simulink model "openMHA_test_FFT_to_gain"  (R2020b)
settings: Solver=VariableStepAuto  StartTime=0.0  StopTime=stop_time  RelTol=1e-3
InitFcn:
  | test_FFT_to_gain_init
StopFcn:
  | test_FFT_to_gain_stop
values from neighbouring files (symbols this model uses):
  band_edges = [band_edges mirrored_band_edges]    [test_FFT_to_gain_init.m]    (also in test_db_lookup_gain_fpga_init.m = calculate_band_edges(ef, num_bins, binwidth, num_bands); test_db_lookup_init.m = calculate_band_edges(ef, num_bins, binwidth, num_bands); test_gaintable_init.m = calculate_band_edges(ef, num_bins, binwidth, num_bands); test_init.m = calculate_band_edges(ef, num_bins, binwidth, num_bands))
  buf_a = 65.*ones(num_bands,1)    [test_FFT_to_gain_init.m]    (also in test_ar_filter_dualport_init.m; test_db_ar_gaintable_init.m)
  delay_memory_size = 2^system_delay_memory    [test_FFT_to_gain_init.m]    (also in test_state_gainapp_cbuf_init.m)
  FFTsize = 256    [test_FFT_to_gain_init.m]    (also in test_ar_filter_gaintable_init.m; test_db_ar_gaintable_init.m; test_db_lookup_gain_fpga_init.m; test_db_lookup_init.m)
  gainapp_dp_memory = log2(num_bands) + 1    [test_FFT_to_gain_init.m]    (also in test_state_gainapp_cbuf_init.m)
  num_bands = 8    [calculate_gaintable.m]    (also in test_FFT_to_gain_init.m = 2; test_ar_filter_dualport_init.m = 2; test_db_ar_gaintable_init.m = 2; test_db_lookup_gain_fpga_init.m = 9)
  num_bins = FFTsize/2 + 1    (= 129)    [test_FFT_to_gain_init.m]    (also in test_ar_filter_gaintable_init.m; test_db_ar_gaintable_init.m; test_db_lookup_gain_fpga_init.m; test_db_lookup_init.m)
  system_delay = 6 + max(band_sizes)    [test_FFT_to_gain_init.m]    (also in test_state_gainapp_cbuf_init.m = max(band_sizes))
  table_length = length(gtdata)    [calculate_gaintable.m]    (also in test_FFT_to_gain_init.m; test_ar_filter_gaintable_init.m; test_db_ar_gaintable_init.m; test_db_lookup_gain_fpga_init.m)
  X_high = 93    [test_FFT_to_gain_init.m]    (also in test_ar_filter_gaintable_init.m = 95; test_db_ar_gaintable_init.m; test_db_lookup_gain_fpga_init.m = 95; test_db_lookup_init.m = 95)
  xIn = [4.65661287308e-10 5.23868948221e-10 5.82076609135e-10 6.40284270048e-10 6.98491930962e-10 7.56699591875e-10 8.14907252789e-10 8.73114913702e-10 9.31322574615e-10 1.04773789644e-09 1.16415321827e-09 1.2805685401e-09 ... (256 elements, 1x256)]    [openMHA_test_db_lookup_gain_Programmable Look-Up Table_init.mat]    (also in openMHA_test_db_lookup_gain_Programmable Lookup Table dB_init.mat = [4.65661287308e-10 4.72937244922e-10 4.80213202536e-10 4.874)
libraries: dspsrcs4 x9, hdlsllib x8, simulink x4, FPGA_Open_Speech_Tools x3
(part 1 of 2)
settings Model: Creator=t96f346  LastModifiedBy=t96f346

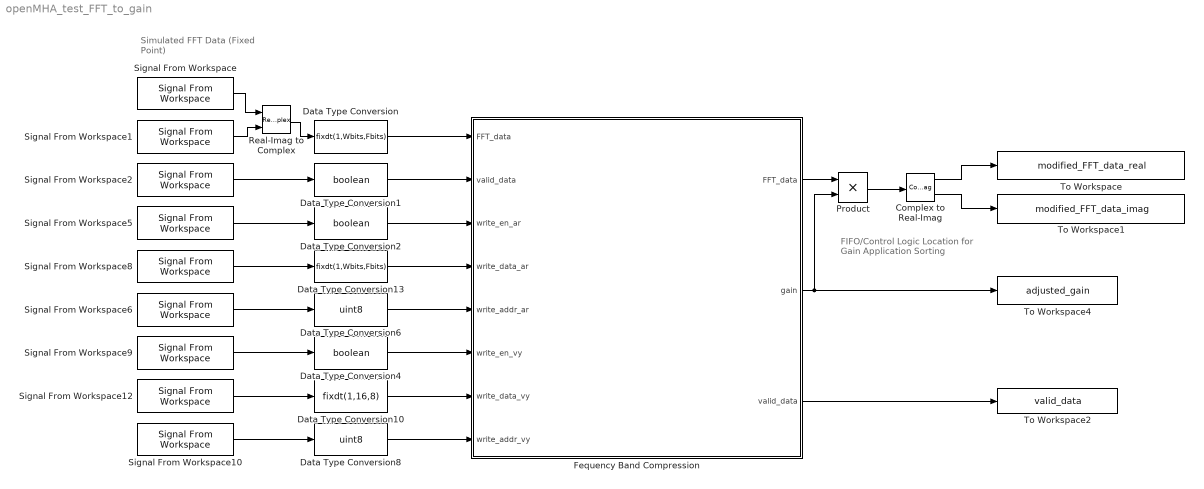
== system openMHA_test_FFT_to_gain ==
  note: Simulated FFT Data
      | (Fixed Point)
  note: FIFO/Control Logic Location for Gain Application Sorting
  Complex to Real-Imag : ComplexToRealImag
  Data Type Conversion : DataTypeConversion  OutDataTypeStr=fixdt(1,Wbits,Fbits)
  Data Type Conversion1 : DataTypeConversion  OutDataTypeStr=boolean
  Data Type Conversion10 : DataTypeConversion  OutDataTypeStr=fixdt(1,16,8)
  Data Type Conversion13 : DataTypeConversion  OutDataTypeStr=fixdt(1,Wbits,Fbits)
  Data Type Conversion2 : DataTypeConversion  OutDataTypeStr=boolean
  Data Type Conversion4 : DataTypeConversion  OutDataTypeStr=boolean
  Data Type Conversion6 : DataTypeConversion  OutDataTypeStr=uint8
  Data Type Conversion8 : DataTypeConversion  OutDataTypeStr=uint8
  Fequency Band Compression : Subsystem
  Product : Product
  Real-Imag to Complex : RealImagToComplex
  Signal From Workspace : dspsrcs4/Signal From Workspace  X=FFT_data_real  Ts=1  nsamps=1  OutputAfterFinalValue=Setting to zero  ignoreOrWarnInputAndFrameLengths=off  OutputFrames=off
  Signal From Workspace1 : dspsrcs4/Signal From Workspace  X=FFT_data_imag  Ts=1  nsamps=1  OutputAfterFinalValue=Setting to zero  ignoreOrWarnInputAndFrameLengths=off  OutputFrames=off
  Signal From Workspace10 : dspsrcs4/Signal From Workspace  X=write_addr_vy  Ts=1  nsamps=1  OutputAfterFinalValue=Setting to zero  ignoreOrWarnInputAndFrameLengths=off  OutputFrames=off
  Signal From Workspace12 : dspsrcs4/Signal From Workspace  X=write_data_vy  Ts=1  nsamps=1  OutputAfterFinalValue=Setting to zero  ignoreOrWarnInputAndFrameLengths=off  OutputFrames=off
  Signal From Workspace2 : dspsrcs4/Signal From Workspace  X=valid_data  Ts=1  nsamps=1  OutputAfterFinalValue=Setting to zero  ignoreOrWarnInputAndFrameLengths=off  OutputFrames=off
  Signal From Workspace5 : dspsrcs4/Signal From Workspace  X=write_en_ar  Ts=1  nsamps=1  OutputAfterFinalValue=Setting to zero  ignoreOrWarnInputAndFrameLengths=off  OutputFrames=off
  Signal From Workspace6 : dspsrcs4/Signal From Workspace  X=write_addr_ar  Ts=1  nsamps=1  OutputAfterFinalValue=Setting to zero  ignoreOrWarnInputAndFrameLengths=off  OutputFrames=off
  Signal From Workspace8 : dspsrcs4/Signal From Workspace  X=write_data_ar  Ts=1  nsamps=1  OutputAfterFinalValue=Setting to zero  ignoreOrWarnInputAndFrameLengths=off  OutputFrames=off
  Signal From Workspace9 : dspsrcs4/Signal From Workspace  X=write_en_vy  Ts=1  nsamps=1  OutputAfterFinalValue=Setting to zero  ignoreOrWarnInputAndFrameLengths=off  OutputFrames=off
  To Workspace : ToWorkspace  VariableName=modified_FFT_data_real  SampleTime=-1
      settings: Save2DSignal=2-D array (concatenate along first dimension)
  To Workspace1 : ToWorkspace  VariableName=modified_FFT_data_imag  SampleTime=-1
      settings: Save2DSignal=2-D array (concatenate along first dimension)
  To Workspace2 : ToWorkspace  VariableName=valid_data  SampleTime=-1
      settings: Save2DSignal=2-D array (concatenate along first dimension)
  To Workspace4 : ToWorkspace  VariableName=adjusted_gain  SampleTime=-1
      settings: Save2DSignal=2-D array (concatenate along first dimension)
  wires:
  Real-Imag to Complex/1 -> Data Type Conversion/1
  Signal From Workspace1/1 -> Real-Imag to Complex/2
  Signal From Workspace/1 -> Real-Imag to Complex/1
  Product/1 -> Complex to Real-Imag/1
  Complex to Real-Imag/2 -> To Workspace1/1
  Complex to Real-Imag/1 -> To Workspace/1
  Data Type Conversion/1 -> Fequency Band Compression/1(FFT_data)
  Signal From Workspace2/1 -> Data Type Conversion1/1
  Signal From Workspace12/1 -> Data Type Conversion10/1
  Signal From Workspace8/1 -> Data Type Conversion13/1
  Signal From Workspace10/1 -> Data Type Conversion8/1
  Signal From Workspace9/1 -> Data Type Conversion4/1
  Signal From Workspace6/1 -> Data Type Conversion6/1
  Signal From Workspace5/1 -> Data Type Conversion2/1
  Data Type Conversion2/1 -> Fequency Band Compression/3(write_en_ar)
  Data Type Conversion13/1 -> Fequency Band Compression/4(write_data_ar)
  Data Type Conversion6/1 -> Fequency Band Compression/5(write_addr_ar)
  Data Type Conversion4/1 -> Fequency Band Compression/6(write_en_vy)
  Data Type Conversion10/1 -> Fequency Band Compression/7(write_data_vy)
  Data Type Conversion8/1 -> Fequency Band Compression/8(write_addr_vy)
  Fequency Band Compression/2(gain) -> Product/2, To Workspace4/1
  Data Type Conversion1/1 -> Fequency Band Compression/2(valid_data)
  Fequency Band Compression/1("FFT_data ") -> Product/1
  Fequency Band Compression/3("valid_data ") -> To Workspace2/1

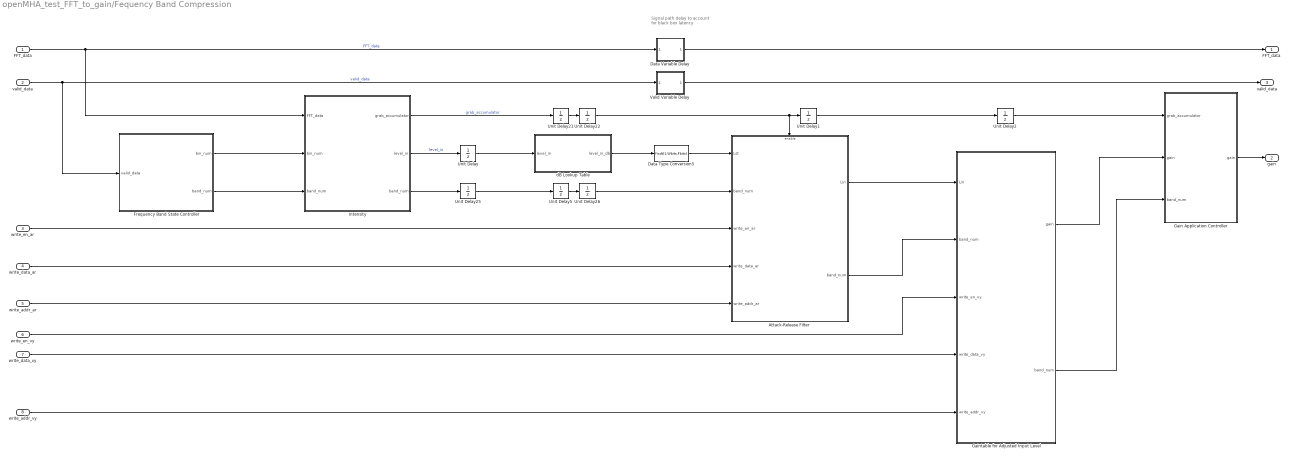
== system openMHA_test_FFT_to_gain/Fequency Band Compression ==
  note: Signal path delay to account for black box latency
  FFT_data : Inport
  valid_data : Inport  Port=2
  write_en_ar : Inport  Port=3
  write_data_ar : Inport  Port=4
  write_addr_ar : Inport  Port=5
  write_en_vy : Inport  Port=6
  write_data_vy : Inport  Port=7
  write_addr_vy : Inport  Port=8
  Attack-Release Filter : Subsystem
  Data Type Conversion5 : DataTypeConversion  OutDataTypeStr=fixdt(1,Wbits,Fbits)
  Data Variable Delay : Subsystem
  Frequency Band State Controller : Subsystem
  Gain Application Controller : Subsystem
  Gaintable for Adjusted Input Level : Subsystem
  Intensity : Subsystem
  Unit Delay{,1..2,5,21..22,25..26} (8 alike) : UnitDelay  SampleTime=-1  HasFrameUpgradeWarning=on
  Valid Variable Delay : Subsystem
  dB Lookup Table : Subsystem
  "FFT_data " : Outport
  gain : Outport  Port=2
  "valid_data " : Outport  Port=3
  wires:
  Gaintable for Adjusted Input Level/1(gain) -> Gain Application Controller/2(gain)
  Intensity/2(level_in) -> Unit Delay/1  "level_in"
  valid_data/1 -> Valid Variable Delay/1(data_in), Frequency Band State Controller/1(valid_data)  "valid_data"
  Intensity/1(grab_accumulator) -> Unit Delay21/1  "grab_accumulator"
  FFT_data/1 -> Data Variable Delay/1(data_in), Intensity/1(FFT_data)  "FFT_data"
  Intensity/3("band_num ") -> Unit Delay25/1
  Unit Delay25/1 -> Unit Delay5/1
  Valid Variable Delay/1(rd_dout) -> "valid_data "/1
  Data Variable Delay/1(rd_dout) -> "FFT_data "/1
  Data Type Conversion5/1 -> Attack-Release Filter/1(Lst)
  dB Lookup Table/1(level_in_db) -> Data Type Conversion5/1
  Unit Delay/1 -> dB Lookup Table/1(level_in)
  Unit Delay5/1 -> Unit Delay26/1
  Unit Delay26/1 -> Attack-Release Filter/2(band_num)
  Attack-Release Filter/1(Lin) -> Gaintable for Adjusted Input Level/1(Lin)
  Attack-Release Filter/2("band_num ") -> Gaintable for Adjusted Input Level/2(band_num)
  Frequency Band State Controller/1(bin_num) -> Intensity/2(bin_num)
  Frequency Band State Controller/2(band_num) -> Intensity/3(band_num)
  Unit Delay21/1 -> Unit Delay22/1
  Unit Delay22/1 -> Attack-Release Filter/Enable, Unit Delay1/1
  write_en_ar/1 -> Attack-Release Filter/3(write_en_ar)
  write_data_ar/1 -> Attack-Release Filter/4(write_data_ar)
  write_addr_ar/1 -> Attack-Release Filter/5(write_addr_ar)
  write_en_vy/1 -> Gaintable for Adjusted Input Level/3(write_en_vy)
  write_data_vy/1 -> Gaintable for Adjusted Input Level/4(write_data_vy)
  write_addr_vy/1 -> Gaintable for Adjusted Input Level/5(write_addr_vy)
  Gaintable for Adjusted Input Level/2("band_num ") -> Gain Application Controller/3(band_num)
  Unit Delay1/1 -> Unit Delay2/1
  Unit Delay2/1 -> Gain Application Controller/1(grab_accumulator)
  Gain Application Controller/1("gain ") -> gain/1

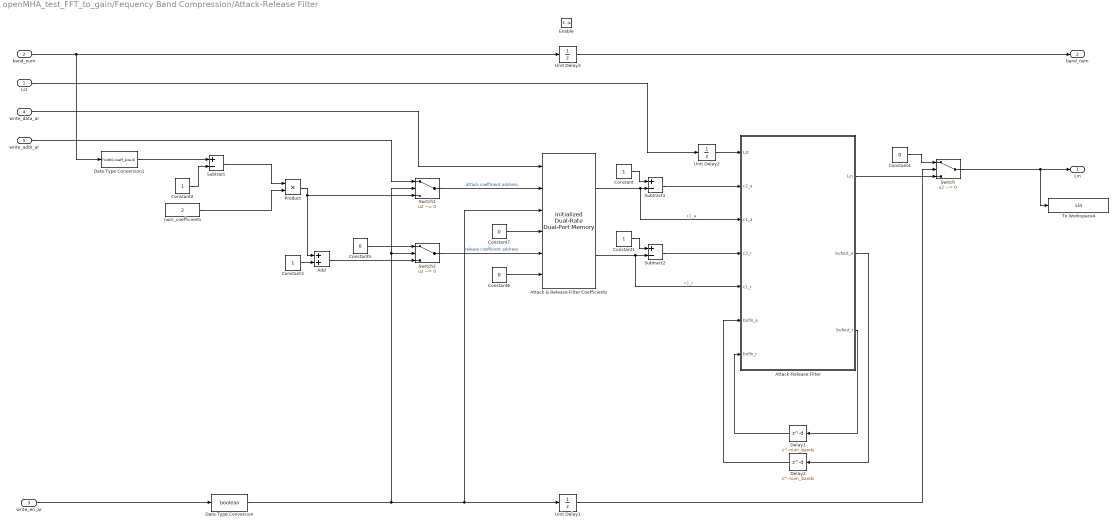
== system openMHA_test_FFT_to_gain/Fequency Band Compression/Attack-Release Filter ==
  Lst : Inport
  band_num : Inport  Port=2
  write_en_ar : Inport  Port=3
  write_data_ar : Inport  Port=4
  write_addr_ar : Inport  Port=5
  Enable : EnablePort
  Add : Sum
  Attack & Release Filter Coefficients : FPGA_Open_Speech_Tools/Initialized Dual-Rate Dual-Port Memory  ram_size=coeff_size  Table_Init=ar_coeffs
      settings: SourceProductName=FPGA Open Speech Tools
  Attack-Release Filter : Subsystem
  Constant : Constant  OutDataTypeStr=fixdt(1,Wbits,Fbits)  SampleTime=-1
  Constant1 : Constant  OutDataTypeStr=fixdt(1,Wbits,Fbits)  SampleTime=-1
  Constant2 : Constant  OutDataTypeStr=fixdt(0,coeff_size,0)  SampleTime=-1
  Constant3 : Constant  OutDataTypeStr=uint8  SampleTime=-1
  Constant4 : Constant  Value=0  OutDataTypeStr=fixdt(1,Wbits,Fbits)  SampleTime=-1
  Constant5 : Constant  Value=0  OutDataTypeStr=uint8  SampleTime=-1
  Constant6 : Constant  Value=0  OutDataTypeStr=boolean  SampleTime=-1
  Constant7 : Constant  Value=0  OutDataTypeStr=fixdt(1,Wbits,Fbits)  SampleTime=-1
  Data Type Conversion : DataTypeConversion  OutDataTypeStr=boolean
  Data Type Conversion1 : DataTypeConversion  OutDataTypeStr=fixdt(0,coeff_size,0)
  Delay1 : Delay  DelayLength=num_bands  InitialCondition=buf_a  UseCircularBuffer=on
  Delay2 : Delay  DelayLength=num_bands  InitialCondition=buf_a  UseCircularBuffer=on
  Product : Product  OutDataTypeStr=fixdt(0,coeff_size,0)
  Subtract : Sum  Inputs=+-  OutDataTypeStr=fixdt(0,coeff_size,0)
  Subtract1 : Sum  Inputs=+-  OutDataTypeStr=fixdt(1,Wbits,Fbits)
  Subtract2 : Sum  Inputs=+-  OutDataTypeStr=fixdt(1,Wbits,Fbits)
  Switch : Switch  Criteria=u2 ~= 0  OutDataTypeStr=fixdt(1,Wbits,Fbits)
  Switch1 : Switch  Criteria=u2 ~= 0  OutDataTypeStr=Inherit: Inherit via back propagation
  Switch2 : Switch  Criteria=u2 ~= 0  OutDataTypeStr=uint8
  To Workspace4 : ToWorkspace  VariableName=Lin  SampleTime=-1
      settings: Save2DSignal=2-D array (concatenate along first dimension)
  Unit Delay1 : UnitDelay  SampleTime=-1  HasFrameUpgradeWarning=on
  Unit Delay2 : UnitDelay  InitialCondition=65  SampleTime=-1  HasFrameUpgradeWarning=on
  Unit Delay3 : UnitDelay  InitialCondition=1  SampleTime=-1  HasFrameUpgradeWarning=on
  num_coefficients : Constant  Value=2  OutDataTypeStr=uint8  SampleTime=-1
  Lin : Outport
  "band_num " : Outport  Port=2
  wires:
  Constant4/1 -> Switch/1
  Constant2/1 -> Subtract/2
  Attack-Release Filter/2(bufout_a) -> Delay2/1
  Delay1/1 -> Attack-Release Filter/7(bufin_r)
  Constant6/1 -> Attack & Release Filter Coefficients/6
  Constant3/1 -> Add/2
  Switch1/1 -> Attack & Release Filter Coefficients/2  "attack coefficient address"
  Constant5/1 -> Switch2/1
  Subtract1/1 -> Attack-Release Filter/2(c2_a)
  num_coefficients/1 -> Product/2
  Attack & Release Filter Coefficients/2 -> Attack-Release Filter/5(c1_r), Subtract2/2  "c1_r"
  Constant7/1 -> Attack & Release Filter Coefficients/4
  Attack-Release Filter/1(Lin) -> Switch/3
  Subtract/1 -> Product/1
  Unit Delay2/1 -> Attack-Release Filter/1(Lst)
  Data Type Conversion1/1 -> Subtract/1
  Constant/1 -> Subtract1/1
  Constant1/1 -> Subtract2/1
  Switch2/1 -> Attack & Release Filter Coefficients/5  "release coefficient address"
  Product/1 -> Add/1, Switch1/3
  Data Type Conversion/1 -> Switch1/2, Switch2/2, Unit Delay1/1, Attack & Release Filter Coefficients/3
  Unit Delay1/1 -> Switch/2
  Subtract2/1 -> Attack-Release Filter/4(c2_r)
  Attack-Release Filter/3(bufout_r) -> Delay1/1
  Delay2/1 -> Attack-Release Filter/6(bufin_a)
  Add/1 -> Switch2/3
  Attack & Release Filter Coefficients/1 -> Attack-Release Filter/3(c1_a), Subtract1/2  "c1_a"
  band_num/1 -> Data Type Conversion1/1, Unit Delay3/1
  Lst/1 -> Unit Delay2/1
  write_data_ar/1 -> Attack & Release Filter Coefficients/1
  write_addr_ar/1 -> Switch1/1
  Switch/1 -> To Workspace4/1, Lin/1
  Unit Delay3/1 -> "band_num "/1
  write_en_ar/1 -> Data Type Conversion/1

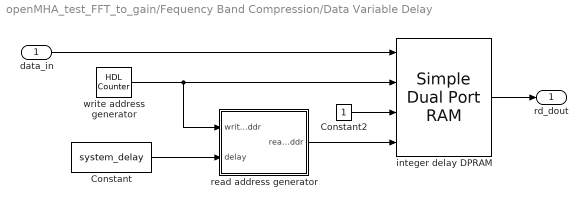
== system openMHA_test_FFT_to_gain/Fequency Band Compression/Data Variable Delay ==
  data_in : Inport
  Constant : Constant  Value=system_delay  OutDataTypeStr=uint8  SampleTime=-1
  Constant2 : Constant  OutDataTypeStr=Inherit: Inherit via back propagation  SampleTime=-1
  integer delay DPRAM : hdlsllib/HDL RAMs/Simple Dual Port RAM  ram_size=system_delay_memory
      settings: SourceProductBaseCode=SL
  read address generator : Subsystem
  write address generator : hdlsllib/Sources/HDL Counter  CountType=Count limited  CountInit=0  CountStep=1  CountMax=delay_memory_size - 1  CountFromType=Initial value  CountFrom=0  CountResetPort=off  CountLoadPort=off  CountEnbPort=off  CountDirPort=off  CountDataType=Unsigned  CountWordLen=system_delay_memory  CountFracLen=0  CountSampTime=-1
  rd_dout : Outport
  wires:
  Constant2/1 -> integer delay DPRAM/3
  write address generator/1 -> integer delay DPRAM/2, read address generator/1(write_addr)
  integer delay DPRAM/1 -> rd_dout/1
  Constant/1 -> read address generator/2(delay)
  data_in/1 -> integer delay DPRAM/1
  read address generator/1(read_addr) -> integer delay DPRAM/4

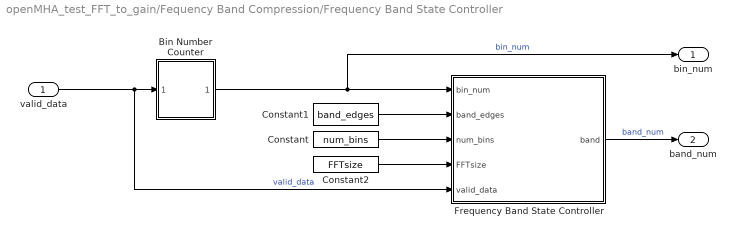
== system openMHA_test_FFT_to_gain/Fequency Band Compression/Frequency Band State Controller ==
  valid_data : Inport
  Bin Number Counter : Subsystem
  Constant : Constant  Value=num_bins  SampleTime=-1
  Constant1 : Constant  Value=band_edges  SampleTime=-1
  Constant2 : Constant  Value=FFTsize  SampleTime=-1
  Frequency Band State Controller : MATLAB Function  TreatAsAtomicUnit=on
  bin_num : Outport
  band_num : Outport  Port=2
  wires:
  Bin Number Counter/1(bin_num) -> bin_num/1, Frequency Band State Controller/1(bin_num)  "bin_num"
  Constant2/1 -> Frequency Band State Controller/4(FFTsize)
  valid_data/1 -> Frequency Band State Controller/5(valid_data), Bin Number Counter/1(valid_data)  "valid_data"
  Constant/1 -> Frequency Band State Controller/3(num_bins)
  Constant1/1 -> Frequency Band State Controller/2(band_edges)
  Frequency Band State Controller/1(band) -> band_num/1  "band_num"

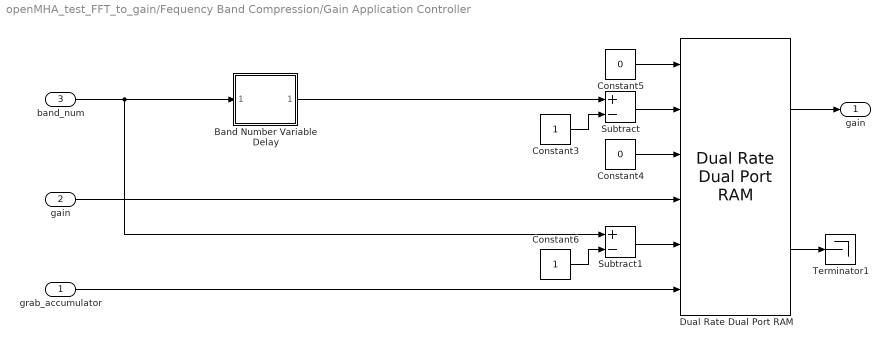
== system openMHA_test_FFT_to_gain/Fequency Band Compression/Gain Application Controller ==
  grab_accumulator : Inport
  gain : Inport  Port=2
  band_num : Inport  Port=3
  Band Number Variable Delay : Subsystem
  Constant3 : Constant  SampleTime=-1
  Constant4 : Constant  Value=0  OutDataTypeStr=boolean  SampleTime=-1
  Constant5 : Constant  Value=0  OutDataTypeStr=fixdt(1,16,8)  SampleTime=-1
  Constant6 : Constant  SampleTime=-1
  Dual Rate Dual Port RAM : hdlsllib/HDL RAMs/Dual Rate Dual Port RAM  ram_size=gainapp_dp_memory
      settings: SourceProductBaseCode=SL
  Subtract : Sum  Inputs=+-  OutMin=[0]  OutMax=[2^gainapp_dp_memory-1]  OutDataTypeStr=fixdt(0,gainapp_dp_memory)
  Subtract1 : Sum  Inputs=+-  OutMin=[0]  OutMax=[2^gainapp_dp_memory-1]  OutDataTypeStr=fixdt(0,gainapp_dp_memory)
  Terminator1 : Terminator
  "gain " : Outport
  wires:
  Dual Rate Dual Port RAM/1 -> "gain "/1
  Constant5/1 -> Dual Rate Dual Port RAM/1
  Constant6/1 -> Subtract1/2
  Constant3/1 -> Subtract/2
  Constant4/1 -> Dual Rate Dual Port RAM/3
  grab_accumulator/1 -> Dual Rate Dual Port RAM/6
  Subtract1/1 -> Dual Rate Dual Port RAM/5
  Band Number Variable Delay/1(rd_dout) -> Subtract/1
  Dual Rate Dual Port RAM/2 -> Terminator1/1
  gain/1 -> Dual Rate Dual Port RAM/4
  Subtract/1 -> Dual Rate Dual Port RAM/2
  band_num/1 -> Band Number Variable Delay/1(data_in), Subtract1/1

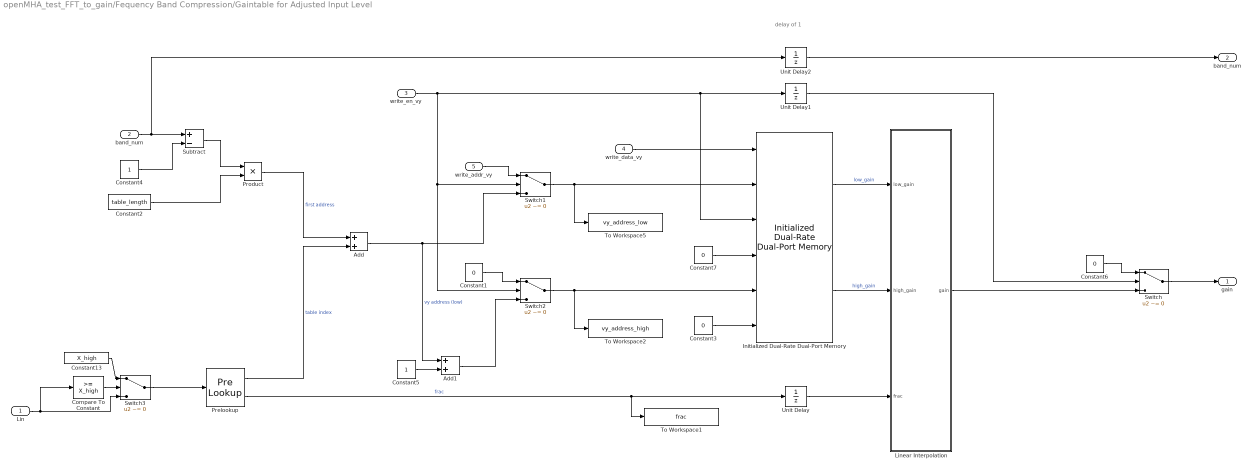
== system openMHA_test_FFT_to_gain/Fequency Band Compression/Gaintable for Adjusted Input Level ==
  note: delay of 1
  Lin : Inport
  band_num : Inport  Port=2
  write_en_vy : Inport  Port=3
  write_data_vy : Inport  Port=4
  write_addr_vy : Inport  Port=5
  Add : Sum  OutDataTypeStr=uint8
  Add1 : Sum  OutDataTypeStr=uint8
  Compare To Constant : simulink/Logic and Bit Operations/Compare To Constant  relop=>=  const=X_high  OutDataTypeStr=boolean
  Constant1 : Constant  Value=0  OutDataTypeStr=uint8  SampleTime=-1
  Constant13 : Constant  Value=X_high  OutDataTypeStr=fixdt(1,Wbits, Fbits)  SampleTime=-1
  Constant2 : Constant  Value=table_length  OutDataTypeStr=uint8  SampleTime=-1
  Constant3 : Constant  Value=0  OutDataTypeStr=boolean  SampleTime=-1
  Constant4 : Constant  OutDataTypeStr=uint8  SampleTime=-1
  Constant5 : Constant  OutDataTypeStr=uint8  SampleTime=-1
  Constant6 : Constant  Value=0  OutDataTypeStr=fixdt(1,16,8)  SampleTime=-1
  Constant7 : Constant  Value=0  OutDataTypeStr=fixdt(1,16,8)  SampleTime=-1
  Initialized Dual-Rate Dual-Port Memory : FPGA_Open_Speech_Tools/Initialized Dual-Rate Dual-Port Memory  ram_size=RAM_size  Table_Init=vy
      settings: SourceProductName=FPGA Open Speech Tools
  Linear Interpolation : Subsystem
  Prelookup : PreLookup  BreakpointsData=input_levels_db  IndexSearchMethod=Evenly spaced points  UseLastBreakpoint=on  DiagnosticForOutOfRangeInput=Error  IndexDataTypeStr=uint8
  Product : Product  OutDataTypeStr=Inherit: Same as first input
  Subtract : Sum  Inputs=+-
  Switch : Switch  Criteria=u2 ~= 0  OutDataTypeStr=fixdt(1,16,8)
  Switch1 : Switch  Criteria=u2 ~= 0  OutDataTypeStr=uint8
  Switch2 : Switch  Criteria=u2 ~= 0  OutDataTypeStr=uint8
  Switch3 : Switch  Criteria=u2 ~= 0
  To Workspace1 : ToWorkspace  VariableName=frac  SampleTime=-1
      settings: Save2DSignal=2-D array (concatenate along first dimension)
  To Workspace2 : ToWorkspace  VariableName=vy_address_high  SampleTime=-1
      settings: Save2DSignal=2-D array (concatenate along first dimension)
  To Workspace5 : ToWorkspace  VariableName=vy_address_low  SampleTime=-1
      settings: Save2DSignal=2-D array (concatenate along first dimension)
  Unit Delay : UnitDelay  SampleTime=-1  HasFrameUpgradeWarning=on
  Unit Delay1 : UnitDelay  InitialCondition=1  SampleTime=-1  HasFrameUpgradeWarning=on
  Unit Delay2 : UnitDelay  InitialCondition=1  SampleTime=-1  HasFrameUpgradeWarning=on
  gain : Outport
  "band_num " : Outport  Port=2
  wires:
  write_data_vy/1 -> Initialized Dual-Rate Dual-Port Memory/1
  Unit Delay/1 -> Linear Interpolation/3(frac)
  Unit Delay1/1 -> Switch/2
  Compare To Constant/1 -> Switch3/2
  Switch/1 -> gain/1
  band_num/1 -> Unit Delay2/1, Subtract/1
  Constant6/1 -> Switch/1
  Add/1 -> Switch1/3, Add1/1  "vy address (low)"
  Linear Interpolation/1(gain) -> Switch/3
  Initialized Dual-Rate Dual-Port Memory/2 -> Linear Interpolation/2(high_gain)  "high_gain"
  Switch1/1 -> Initialized Dual-Rate Dual-Port Memory/2, To Workspace5/1
  write_en_vy/1 -> Initialized Dual-Rate Dual-Port Memory/3, Unit Delay1/1, Switch1/2, Switch2/2
  Constant5/1 -> Add1/2
  Prelookup/1 -> Add/2  "table index"
  Constant13/1 -> Switch3/1
  Add1/1 -> Switch2/3
  Initialized Dual-Rate Dual-Port Memory/1 -> Linear Interpolation/1(low_gain)  "low_gain"
  Switch2/1 -> Initialized Dual-Rate Dual-Port Memory/5, To Workspace2/1
  Constant4/1 -> Subtract/2
  Prelookup/2 -> To Workspace1/1, Unit Delay/1  "frac"
  Product/1 -> Add/1  "first address"
  Subtract/1 -> Product/1
  Lin/1 -> Compare To Constant/1, Switch3/3
  Constant2/1 -> Product/2
  Switch3/1 -> Prelookup/1
  write_addr_vy/1 -> Switch1/1
  Constant1/1 -> Switch2/1
  Constant3/1 -> Initialized Dual-Rate Dual-Port Memory/6
  Constant7/1 -> Initialized Dual-Rate Dual-Port Memory/4
  Unit Delay2/1 -> "band_num "/1

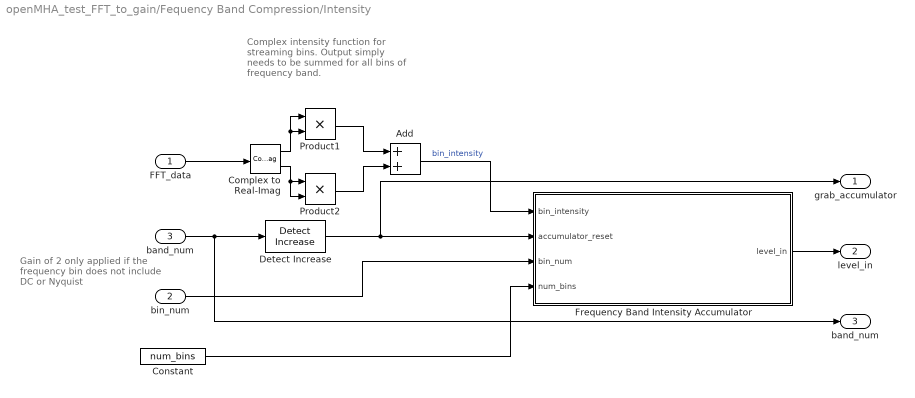
== system openMHA_test_FFT_to_gain/Fequency Band Compression/Intensity ==
  note: Complex intensity function for streaming bins. Output simply needs to be summed for all bins of frequency band.
  note: Gain of 2 only applied if the frequency bin does not include DC or Nyquist
  FFT_data : Inport
  bin_num : Inport  Port=2
  band_num : Inport  Port=3
  Add : Sum  OutDataTypeStr=fixdt(1,Wbits,Fbits)
  Complex to Real-Imag : ComplexToRealImag
  Constant : Constant  Value=num_bins  OutDataTypeStr=uint8  SampleTime=-1
  Detect Increase : simulink/Logic and Bit Operations/Detect Increase  vinit=1  OutDataTypeStr=boolean
  Frequency Band Intensity Accumulator : MATLAB Function  TreatAsAtomicUnit=on
  Product1 : Product  OutDataTypeStr=fixdt(1,Wbits,Fbits)
  Product2 : Product  OutDataTypeStr=fixdt(1,Wbits,Fbits)
  grab_accumulator : Outport  VectorParamsAs1DForOutWhenUnconnected=off
  level_in : Outport  Port=2
  "band_num " : Outport  Port=3
  wires:
  Product2/1 -> Add/2
  Complex to Real-Imag/1 -> Product1/1, Product1/2
  Complex to Real-Imag/2 -> Product2/2, Product2/1
  Product1/1 -> Add/1
  Add/1 -> Frequency Band Intensity Accumulator/1(bin_intensity)  "bin_intensity"
  FFT_data/1 -> Complex to Real-Imag/1
  Frequency Band Intensity Accumulator/1(level_in) -> level_in/1
  band_num/1 -> Detect Increase/1, "band_num "/1
  Detect Increase/1 -> Frequency Band Intensity Accumulator/2(accumulator_reset), grab_accumulator/1
  bin_num/1 -> Frequency Band Intensity Accumulator/3(bin_num)
  Constant/1 -> Frequency Band Intensity Accumulator/4(num_bins)

== system openMHA_test_FFT_to_gain/Fequency Band Compression/Valid Variable Delay ==
  data_in : Inport
  Constant : Constant  Value=system_delay  OutDataTypeStr=uint8  SampleTime=-1
  Constant2 : Constant  OutDataTypeStr=Inherit: Inherit via back propagation  SampleTime=-1
  integer delay DPRAM : hdlsllib/HDL RAMs/Simple Dual Port RAM  ram_size=system_delay_memory
      settings: SourceProductBaseCode=SL
  read address generator : Subsystem
  write address generator : hdlsllib/Sources/HDL Counter  CountType=Count limited  CountInit=0  CountStep=1  CountMax=delay_memory_size - 1  CountFromType=Initial value  CountFrom=0  CountResetPort=off  CountLoadPort=off  CountEnbPort=off  CountDirPort=off  CountDataType=Unsigned  CountWordLen=system_delay_memory  CountFracLen=0  CountSampTime=-1
  rd_dout : Outport
  wires:
  Constant2/1 -> integer delay DPRAM/3
  write address generator/1 -> integer delay DPRAM/2, read address generator/1(write_addr)
  integer delay DPRAM/1 -> rd_dout/1
  Constant/1 -> read address generator/2(delay)
  data_in/1 -> integer delay DPRAM/1
  read address generator/1(read_addr) -> integer delay DPRAM/4

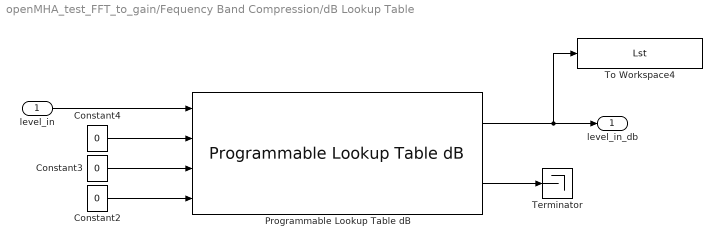
== system openMHA_test_FFT_to_gain/Fequency Band Compression/dB Lookup Table ==
  level_in : Inport
  Constant2 : Constant  Value=0  OutDataTypeStr=boolean  SampleTime=-1
  Constant3 : Constant  Value=0  OutDataTypeStr=uint16  SampleTime=-1
  Constant4 : Constant  Value=0  OutDataTypeStr=fixdt(1,40,32)  SampleTime=-1
  Programmable Lookup Table dB : FPGA_Open_Speech_Tools/Programmable Lookup Table dB  tableFnParam=10.*log10(2500000000.*xIn)  SAVE_TABLE=off  maxInput=1  floorParam=2^-31  errorParam=1  ERR_DIAG=on  PLOT_TABLE=off  nBitsParam=5  mBitsParam=4  IGOTTHIS=off  W_bits=40  F_bits=37  tableInit=0  binaryOffset=0
      link override High_LUT/ram_data: InitialCondition=55.36
      link override Linear_Approximation/Unit Delay: InitialCondition=65
      link override LogAddressing/Delay1: InitialCondition=13
      link override LogAddressing/Delay2: InitialCondition=0.0001265
      link override Low_LUT/ram_data: InitialCondition=54.85
      link override Unit Delay1: InitialCondition=0.0001265
      link override Unit Delay2: InitialCondition=0.0001265
      link override Unit Delay3: InitialCondition=144
      settings: SourceProductName=FPGA Open Speech Tools
  Terminator : Terminator
  To Workspace4 : ToWorkspace  VariableName=Lst  SampleTime=-1
      settings: Save2DSignal=2-D array (concatenate along first dimension)
  level_in_db : Outport
  wires:
  Programmable Lookup Table dB/2 -> Terminator/1
  level_in/1 -> Programmable Lookup Table dB/1
  Programmable Lookup Table dB/1 -> To Workspace4/1, level_in_db/1
  Constant4/1 -> Programmable Lookup Table dB/2
  Constant3/1 -> Programmable Lookup Table dB/3
  Constant2/1 -> Programmable Lookup Table dB/4

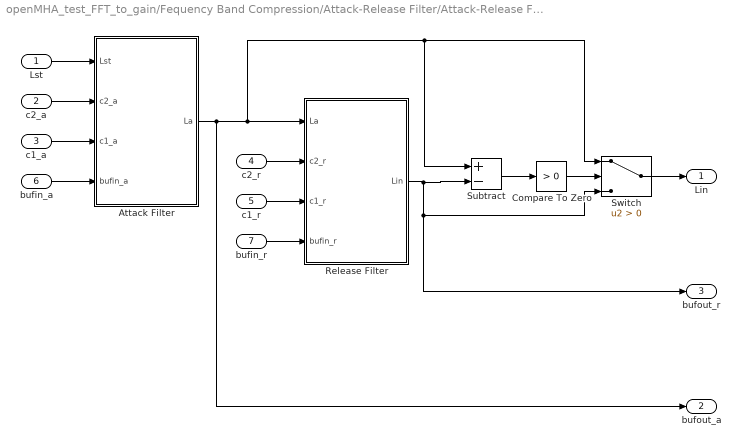
== system openMHA_test_FFT_to_gain/Fequency Band Compression/Attack-Release Filter/Attack-Release Filter ==
  Lst : Inport
  c2_a : Inport  Port=2
  c1_a : Inport  Port=3
  c2_r : Inport  Port=4
  c1_r : Inport  Port=5
  bufin_a : Inport  Port=6
  bufin_r : Inport  Port=7
  Attack Filter : Subsystem  TreatAsAtomicUnit=on
  Compare To Zero : simulink/Logic and Bit Operations/Compare To Zero  relop=>  OutDataTypeStr=boolean
  Release Filter : Subsystem  TreatAsAtomicUnit=on
  Subtract : Sum  Inputs=+-  OutDataTypeStr=fixdt(0,Wbits,Fbits)
  Switch : Switch  Criteria=u2 > Threshold  OutDataTypeStr=fixdt(0,Wbits,Fbits)
  Lin : Outport  VectorParamsAs1DForOutWhenUnconnected=off
  bufout_a : Outport  Port=2  VectorParamsAs1DForOutWhenUnconnected=off
  bufout_r : Outport  Port=3  VectorParamsAs1DForOutWhenUnconnected=off
  wires:
  Lst/1 -> Attack Filter/1(Lst)
  c2_a/1 -> Attack Filter/2(c2_a)
  c1_a/1 -> Attack Filter/3(c1_a)
  bufin_a/1 -> Attack Filter/4(bufin_a)
  c2_r/1 -> Release Filter/2(c2_r)
  c1_r/1 -> Release Filter/3(c1_r)
  bufin_r/1 -> Release Filter/4(bufin_r)
  Attack Filter/1(La) -> bufout_a/1, Switch/1, Subtract/1, Release Filter/1(La)
  Compare To Zero/1 -> Switch/2
  Release Filter/1(Lin) -> Subtract/2, Switch/3, bufout_r/1
  Subtract/1 -> Compare To Zero/1
  Switch/1 -> Lin/1

== system openMHA_test_FFT_to_gain/Fequency Band Compression/Data Variable Delay/read address generator ==
  note: wrap on overflow is the desired behavior
  write_addr : Inport
  delay : Inport  Port=2
  Constant : Constant  Value=delay_memory_size  SampleTime=-1
  Subtract : Sum  Inputs=-++  OutDataTypeStr=Inherit: Inherit via back propagation
  read_addr : Outport  VectorParamsAs1DForOutWhenUnconnected=off
  wires:
  Subtract/1 -> read_addr/1
  write_addr/1 -> Subtract/2
  delay/1 -> Subtract/1
  Constant/1 -> Subtract/3

== system openMHA_test_FFT_to_gain/Fequency Band Compression/Frequency Band State Controller/Bin Number Counter ==
  valid_data : Inport
  Detect Decrease : simulink/Logic and Bit Operations/Detect Decrease  vinit=1  OutDataTypeStr=boolean
  HDL Counter : hdlsllib/Sources/HDL Counter  CountType=Count limited  CountInit=0  CountStep=1  CountMax=FFTsize-1  CountFromType=Initial value  CountFrom=0  CountResetPort=on  CountLoadPort=off  CountEnbPort=on  CountDirPort=off  CountDataType=Unsigned  CountWordLen=log2(FFTsize)  CountFracLen=0  CountSampTime=1
  bin_num : Outport
  wires:
  valid_data/1 -> HDL Counter/2, Detect Decrease/1
  HDL Counter/1 -> bin_num/1
  Detect Decrease/1 -> HDL Counter/1

== system openMHA_test_FFT_to_gain/Fequency Band Compression/Gain Application Controller/Band Number Variable Delay ==
  data_in : Inport
  Constant : Constant  Value=system_delay-6  OutDataTypeStr=uint8  SampleTime=-1
  Constant2 : Constant  OutDataTypeStr=Inherit: Inherit via back propagation  SampleTime=-1
  integer delay DPRAM : hdlsllib/HDL RAMs/Simple Dual Port RAM  ram_size=system_delay_memory
      settings: SourceProductBaseCode=SL
  read address generator : Subsystem
  write address generator : hdlsllib/Sources/HDL Counter  CountType=Count limited  CountInit=0  CountStep=1  CountMax=delay_memory_size-1  CountFromType=Initial value  CountFrom=0  CountResetPort=off  CountLoadPort=off  CountEnbPort=off  CountDirPort=off  CountDataType=Unsigned  CountWordLen=system_delay_memory  CountFracLen=0  CountSampTime=-1
  rd_dout : Outport
  wires:
  Constant2/1 -> integer delay DPRAM/3
  write address generator/1 -> integer delay DPRAM/2, read address generator/1(write_addr)
  integer delay DPRAM/1 -> rd_dout/1
  Constant/1 -> read address generator/2(delay)
  data_in/1 -> integer delay DPRAM/1
  read address generator/1(read_addr) -> integer delay DPRAM/4

== system openMHA_test_FFT_to_gain/Fequency Band Compression/Gaintable for Adjusted Input Level/Linear Interpolation ==
  low_gain : Inport
  high_gain : Inport  Port=2
  frac : Inport  Port=3
  Add : Sum
  Product : Product  OutDataTypeStr=Inherit: Same as first input
  Subtract : Sum  Inputs=-+
  gain : Outport
  wires:
  high_gain/1 -> Subtract/2
  low_gain/1 -> Add/1, Subtract/1
  Subtract/1 -> Product/1
  frac/1 -> Product/2
  Product/1 -> Add/2
  Add/1 -> gain/1

== system openMHA_test_FFT_to_gain/Fequency Band Compression/Valid Variable Delay/read address generator ==
  note: wrap on overflow is the desired behavior
  write_addr : Inport
  delay : Inport  Port=2
  Constant : Constant  Value=delay_memory_size  SampleTime=-1
  Subtract : Sum  Inputs=-++  OutDataTypeStr=Inherit: Inherit via back propagation
  read_addr : Outport  VectorParamsAs1DForOutWhenUnconnected=off
  wires:
  Subtract/1 -> read_addr/1
  write_addr/1 -> Subtract/2
  delay/1 -> Subtract/1
  Constant/1 -> Subtract/3

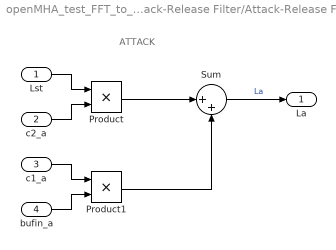
== system openMHA_test_FFT_to_gain/Fequency Band Compression/Attack-Release Filter/Attack-Release Filter/Attack Filter ==
  note: ATTACK
  Lst : Inport
  c2_a : Inport  Port=2
  c1_a : Inport  Port=3
  bufin_a : Inport  Port=4
  Product : Product  OutDataTypeStr=fixdt(0,Wbits,Fbits)
  Product1 : Product  OutDataTypeStr=fixdt(0,Wbits,Fbits)
  Sum : Sum  Inputs=|++  OutDataTypeStr=fixdt(0,Wbits,Fbits)
  La : Outport  InitialOutput=0  VectorParamsAs1DForOutWhenUnconnected=off
  wires:
  Lst/1 -> Product/1
  Product/1 -> Sum/1
  Sum/1 -> La/1  "La"
  bufin_a/1 -> Product1/2
  Product1/1 -> Sum/2
  c2_a/1 -> Product/2
  c1_a/1 -> Product1/1

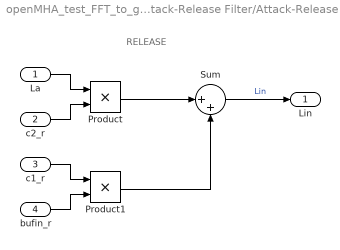
== system openMHA_test_FFT_to_gain/Fequency Band Compression/Attack-Release Filter/Attack-Release Filter/Release Filter ==
  note: RELEASE
  La : Inport
  c2_r : Inport  Port=2
  c1_r : Inport  Port=3
  bufin_r : Inport  Port=4
  Product : Product  OutDataTypeStr=fixdt(0,Wbits,Fbits)
  Product1 : Product  OutDataTypeStr=fixdt(0,Wbits,Fbits)
  Sum : Sum  Inputs=|++  OutDataTypeStr=fixdt(0,Wbits,Fbits)
  Lin : Outport  InitialOutput=0  VectorParamsAs1DForOutWhenUnconnected=off
  wires:
  Sum/1 -> Lin/1  "Lin"
  c2_r/1 -> Product/2
  c1_r/1 -> Product1/1
  La/1 -> Product/1
  Product1/1 -> Sum/2
  Product/1 -> Sum/1
  bufin_r/1 -> Product1/2

== system openMHA_test_FFT_to_gain/Fequency Band Compression/Gain Application Controller/Band Number Variable Delay/read address generator ==
  note: wrap on overflow is the desired behavior
  write_addr : Inport
  delay : Inport  Port=2
  Constant : Constant  Value=delay_memory_size  SampleTime=-1
  Subtract : Sum  Inputs=-++  OutDataTypeStr=Inherit: Inherit via back propagation
  read_addr : Outport  VectorParamsAs1DForOutWhenUnconnected=off
  wires:
  Subtract/1 -> read_addr/1
  write_addr/1 -> Subtract/2
  delay/1 -> Subtract/1
  Constant/1 -> Subtract/3

== matlab function openMHA_test_FFT_to_gain/Fequency Band Compression/Frequency Band State Controller/Frequency Band State Controller ==
  data: bin_num input; band output; band_edges input size=[1 64]; num_bins input; FFTsize input; valid_data input
%#codegen
function band = band_state_controller(bin_num, band_edges, num_bins, FFTsize, valid_data)
% Moore State Machine

%------------------------------------------------------------------------%
% The following is a Moore State Machine in which each state represents the
% frequency band in which the dynamic compression model is operating. The
% frequency bin number or index is the input to the state machine and
% determines whether whether the next state will be in the current, next,
% or previous frequency band. The band_edges input is designed to read 
% from a precomputed band edge index vector, which sets the boundaries 
% between each frequency band and serves as the conditional value.
%------------------------------------------------------------------------%

% y = f(x) : 
% all actions are state actions and 
% outputs are pure functions of state only 

% Defining All Possible Frequency Band States
fb1 = 1;
fb2 = 2;
fb3 = 3;
fb4 = 4;
fb5 = 5;
fb6 = 6;
fb7 = 7;
fb8 = 8;
fb9 = 9;
fb10 = 10;
fb11 = 11;
fb12 = 12;
fb13 = 13;
fb14 = 14;
fb15 = 15;
fb16 = 16;
fb17 = 17;
fb18 = 18;
fb19 = 19;
fb20 = 20;
fb21 = 21;
fb22 = 22;
fb23 = 23;
fb24 = 24;
fb25 = 25;
fb26 = 26;
fb27 = 27;
fb28 = 28;
fb29 = 29;
fb30 = 30;
fb31 = 31;
fb32 = 32;


% Using persistent keyword to model state registers in hardware
persistent curr_state;
if isempty(curr_state)
    curr_state = fb1;   
end

% Switch to new state (frequency band) based on the value state register
switch (curr_state)
    
    case fb1
        
        % value of output band depends only on state and not on inputs
        band = uint8(1);
        
        % decide next state value based on inputs
        if bin_num >= FFTsize-1
            curr_state = fb1;
        elseif bin_num >= num_bins - 1
            curr_state = fb1;
        elseif (bin_num >= band_edges(band)) && (valid_data == true)
            curr_state = fb2;
        else
            curr_state = fb1;
        end
        
        
    case fb2
        
        band = uint8(2);
        
        if bin_num >= FFTsize-1
            curr_state = fb1;
        elseif bin_num >= num_bins-1
            if bin_num >= band_edges(band + (length(band_edges)/2))
                curr_state = fb1;
            else
                curr_state = fb2;
            end
        elseif (bin_num >= band_edges(band))
            curr_state = fb3;
        else
            curr_state = fb2;
        end
        
        
    case fb3
        
        band = uint8(3);
        
        if bin_num >= FFTsize-1
            curr_state = fb1;
        elseif bin_num >= num_bins-1
            if bin_num >= band_edges(band + (length(band_edges)/2))
                curr_state = fb2;
            else
                curr_state = fb3;
            end
        elseif (bin_num >= band_edges(band))
            curr_state = fb4;
        else
            curr_state = fb3;
        end
        

    case fb4
        
        band = uint8(4);
        
        if bin_num >= FFTsize-1
            curr_state = fb1;
        elseif bin_num >= num_bins-1
            if bin_num >= band_edges(band + (length(band_edges)/2))
                curr_state = fb3;
            else
                curr_state = fb4;
            end
        elseif (bin_num >= band_edges(band))
            curr_state = fb5;
        else
            curr_state = fb4;
        end

        
    case fb5
        
        band = uint8(5);
        
        if bin_num >= FFTsize-1
            curr_state = fb1;
        elseif bin_num >= num_bins-1
            if bin_num >= band_edges(band + (length(band_edges)/2))
                curr_state = fb4;
            else
                curr_state = fb5;
            end
        elseif (bin_num >= band_edges(band))
            curr_state = fb6;
        else
            curr_state = fb5;
        end        

        
    case fb6
        
        band = uint8(6);
        
        if bin_num >= FFTsize-1
            curr_state = fb1;
        elseif bin_num >= num_bins-1
            if bin_num >= band_edges(band + (length(band_edges)/2))
                curr_state = fb5;
            else
                curr_state = fb6;
            end
        elseif (bin_num >= band_edges(band))
            curr_state = fb7;
        else
            curr_state = fb6;
        end  
        
        
    case fb7
        
        band = uint8(7);
        
        if bin_num >= FFTsize-1
            curr_state = fb1;
        elseif bin_num >= num_bins-1
            if bin_num >= band_edges(band + (length(band_edges)/2))
                curr_state = fb6;
            else
                curr_state = fb7;
            end
        elseif (bin_num >= band_edges(band))
            curr_state = fb8;
        else
            curr_state = fb7;
        end  
        
        
    case fb8
        
        band = uint8(8);
        
        if bin_num >= FFTsize-1
            curr_state = fb1;
        elseif bin_num >= num_bins-1
            if bin_num >= band_edges(band + (length(band_edges)/2))
                curr_state = fb7;
            else
                curr_state = fb8;
            end
        elseif (bin_num >= band_edges(band))
            curr_state = fb9;
        else
            curr_state = fb8;
        end  
        
        
    case fb9
        
        band = uint8(9);
        
        if bin_num >= FFTsize-1
            curr_state = fb1;
        elseif bin_num >= num_bins-1
            if bin_num >= band_edges(band + (length(band_edges)/2))
                curr_state = fb8;
            else
                curr_state = fb9;
            end
        elseif (bin_num >= band_edges(band))
            curr_state = fb10;
        else
            curr_state = fb9;
        end  
        
        
    case fb10
        
        band = uint8(10);
        
        if bin_num >= FFTsize-1
            curr_state = fb1;
        elseif bin_num >= num_bins-1
            if bin_num >= band_edges(band + (length(band_edges)/2))
                curr_state = fb9;
            else
                curr_state = fb10;
            end
        elseif (bin_num >= band_edges(band))
            curr_state = fb11;
        else
            curr_state = fb10;
        end  
        
        
    case fb11
        
        band = uint8(11);
        
        if bin_num >= FFTsize-1
            curr_state = fb1;
        elseif bin_num >= num_bins-1
            if bin_num >= band_edges(band + (length(band_edges)/2))
                curr_state = fb10;
            else
                curr_state = fb11;
            end
        elseif (bin_num >= band_edges(band))
            curr_state = fb12;
        else
            curr_state = fb11;
        end  
        
        
    case fb12
        
        band = uint8(12);
        
        if bin_num >= FFTsize-1
            curr_state = fb1;
        elseif bin_num >= num_bins-1
            if bin_num >= band_edges(band + (length(band_edges)/2))
                curr_state = fb11;
            else
                curr_state = fb12;
            end
        elseif (bin_num >= band_edges(band))
            curr_state = fb13;
        else
            curr_state = fb12;
        end  
        
        
    case fb13
        
        band = uint8(13);
        
        if bin_num >= FFTsize-1
            curr_state = fb1;
        elseif bin_num >= num_bins-1
            if bin_num >= band_edges(band + (length(band_edges)/2))
                curr_state = fb12;
            else
                curr_state = fb13;
            end
        elseif (bin_num >= band_edges(band))
            curr_state = fb14;
        else
            curr_state = fb13;
        end  
        
        
    case fb14
        
        band = uint8(14);
        
        if bin_num >= FFTsize-1
            curr_state = fb1;
        elseif bin_num >= num_bins-1
            if bin_num >= band_edges(band + (length(band_edges)/2))
                curr_state = fb13;
            else
                curr_state = fb14;
            end
        elseif (bin_num >= band_edges(band))
            curr_state = fb15;
        else
            curr_state = fb14;
        end  
        
        
    case fb15
        
        band = uint8(15);
        
        if bin_num >= FFTsize-1
            curr_state = fb1;
        elseif bin_num >= num_bins-1
            if bin_num >= band_edges(band + (length(band_edges)/2))
                curr_state = fb14;
            else
                curr_state = fb15;
            end
        elseif (bin_num >= band_edges(band))
            curr_state = fb16;
        else
            curr_state = fb15;
        end  
        
        
    case fb16
        
        band = uint8(16);
        
        if bin_num >= FFTsize-1
            curr_state = fb1;
        elseif bin_num >= num_bins-1
            if bin_num >= band_edges(band + (length(band_edges)/2))
                curr_state = fb15;
            else
                curr_state = fb16;
            end
        elseif (bin_num >= band_edges(band))
            curr_state = fb17;
        else
            curr_state = fb16;
        end  
        
        
    case fb17
        
        band = uint8(17);
        
        if bin_num >= FFTsize-1
            curr_state = fb1;
        elseif bin_num >= num_bins-1
            if bin_num >= band_edges(band + (length(band_edges)/2))
                curr_state = fb16;
            else
                curr_state = fb17;
            end
        elseif (bin_num >= band_edges(band))
            curr_state = fb18;
        else
            curr_state = fb17;
        end  
        
        
    case fb18
        
        band = uint8(18);
        
        if bin_num >= FFTsize-1
            curr_state = fb1;
        elseif bin_num >= num_bins-1
            if bin_num >= band_edges(band + (length(band_edges)/2))
                curr_state = fb17;
            else
                curr_state = fb18;
            end
        elseif (bin_num >= band_edges(band))
            curr_state = fb19;
        else
            curr_state = fb18;
        end  
        
        
    case fb19
        
        band = uint8(19);
        
        if bin_num >= FFTsize-1
            curr_state = fb1;
        elseif bin_num >= num_bins-1
            if bin_num >= band_edges(band + (length(band_edges)/2))
                curr_state = fb18;
            else
                curr_state = fb19;
            end
        elseif (bin_num >= band_edges(band))
            curr_state = fb20;
        else
            curr_state = fb19;
        end  
        
        
    case fb20
        
        band = uint8(20);
        
        if bin_num >= FFTsize-1
            curr_state = fb1;
        elseif bin_num >= num_bins-1
            if bin_num >= band_edges(band + (length(band_edges)/2))
                curr_state = fb19;
            else
                curr_state = fb20;
            end
        elseif (bin_num >= band_edges(band))
            curr_state = fb21;
        else
            curr_state = fb20;
        end  
        
        
    case fb21
        
        band = uint8(21);
        
        if bin_num >= FFTsize-1
            curr_state = fb1;
        elseif bin_num >= num_bins-1
            if bin_num >= band_edges(band + (length(band_edges)/2))
                curr_state = fb20;
            else
                curr_state = fb21;
            end
        elseif (bin_num >= band_edges(band))
            curr_state = fb22;
        else
            curr_state = fb21;
        end
        
        
    case fb22
        
        band = uint8(22);
        
        if bin_num >= FFTsize-1
            curr_state = fb1;
        elseif bin_num >= num_bins-1
            if bin_num >= band_edges(band + (length(band_edges)/2))
                curr_state = fb21;
            else
                curr_state = fb22;
            end
        elseif (bin_num >= band_edges(band))
            curr_state = fb23;
        else
            curr_state = fb22;
        end
        
        
    case fb23
        
        band = uint8(23);
        
        if bin_num >= FFTsize-1
            curr_state = fb1;
        elseif bin_num >= num_bins-1
            if bin_num >= band_edges(band + (length(band_edges)/2))
                curr_state = fb22;
            else
                curr_state = fb23;
            end
        elseif (bin_num >= band_edges(band))
            curr_state = fb24;
        else
            curr_state = fb23;
        end
        
        
    case fb24
        
        band = uint8(24);
        
        if bin_num >= FFTsize-1
            curr_state = fb1;
        elseif bin_num >= num_bins-1
            if bin_num >= band_edges(band + (length(band_edges)/2))
                curr_state = fb23;
            else
                curr_state = fb24;
            end
        elseif (bin_num >= band_edges(band))
            curr_state = fb25;
        else
            curr_state = fb24;
        end
        
        
    case fb25
        
        band = uint8(25);
        
        if bin_num >= FFTsize-1
            curr_state = fb1;
        elseif bin_num >= num_bins-1
            if bin_num >= band_edges(band + (length(band_edges)/2))
                curr_state = fb24;
            else
                curr_state = fb25;
            end
        elseif (bin_num >= band_edges(band))
            curr_state = fb26;
        else
            curr_state = fb25;
        end
        
        
    case fb26
        
        band = uint8(26);
        
        if bin_num >= FFTsize-1
            curr_state = fb1;
        elseif bin_num >= num_bins-1
            if bin_num >= band_edges(band + (length(band_edges)/2))
                curr_state = fb25;
            else
                curr_state = fb26;
            end
        elseif (bin_num >= band_edges(band))
            curr_state = fb27;
        else
            curr_state = fb26;
        end
        
        
    case fb27
        
        band = uint8(27);
        
        if bin_num >= FFTsize-1
            curr_state = fb1;
        elseif bin_num >= num_bins-1
            if bin_num >= band_edges(band + (length(band_edges)/2))
                curr_state = fb26;
            else
                curr_state = fb27;
            end
        elseif (bin_num >= band_edges(band))
            curr_state = fb28;
        else
            curr_state = fb27;
        end
        
        
    case fb28
        
        band = uint8(28);
        
        if bin_num >= FFTsize-1
            curr_state = fb1;
        elseif bin_num >= num_bins-1
            if bin_num >= band_edges(band + (length(band_edges)/2))
                curr_state = fb27;
            else
                curr_state = fb28;
            end
        elseif (bin_num >= band_edges(band))
            curr_state = fb29;
        else
            curr_state = fb28;
        end
        
        
    case fb29
        
        band = uint8(29);
        
        if bin_num >= FFTsize-1
            curr_state = fb1;
        elseif bin_num >= num_bins-1
            if bin_num >= band_edges(band + (length(band_edges)/2))
                curr_state = fb28;
            else
                curr_state = fb29;
            end
        elseif (bin_num >= band_edges(band))
            curr_state = fb30;
        else
            curr_state = fb29;
        end
        
        
    case fb30
        
        band = uint8(30);
        
        if bin_num >= FFTsize-1
            curr_state = fb1;
        elseif bin_num >= num_bins-1
            if bin_num >= band_edges(band + (length(band_edges)/2))
                curr_state = fb29;
            else
                curr_state = fb30;
            end
        elseif (bin_num >= band_edges(band))
            curr_state = fb31;
        else
            curr_state = fb30;
        end
        
        
    case fb31
        
        band = uint8(31);
        
        if bin_num >= FFTsize-1
            curr_state = fb1;
        elseif bin_num >= num_bins-1
            if bin_num >= band_edges(band + (length(band_edges)/2))
                curr_state = fb30;
            else
                curr_state = fb31;
            end
        elseif (bin_num >= band_edges(band))
            curr_state = fb32;
        else
            curr_state = fb31;
        end
        
        
    case fb32
        
        band = uint8(32);
        
        if bin_num >= FFTsize-1
            curr_state = fb1;
        elseif bin_num >= num_bins-1
            if bin_num >= band_edges(band + (length(band_edges)/2))
                curr_state = fb31;
            else
                curr_state = fb32;
            end
        else
            curr_state = fb32;
        end
        
    otherwise
        band = uint8(1);
        
end
